simulink model "steady_state_error_test"  (R2017a)
settings: Solver=VariableStepAuto  StartTime=0.0  StopTime=20  RelTol=1e-3
settings Model: Creator=USER  LastModifiedBy=dell

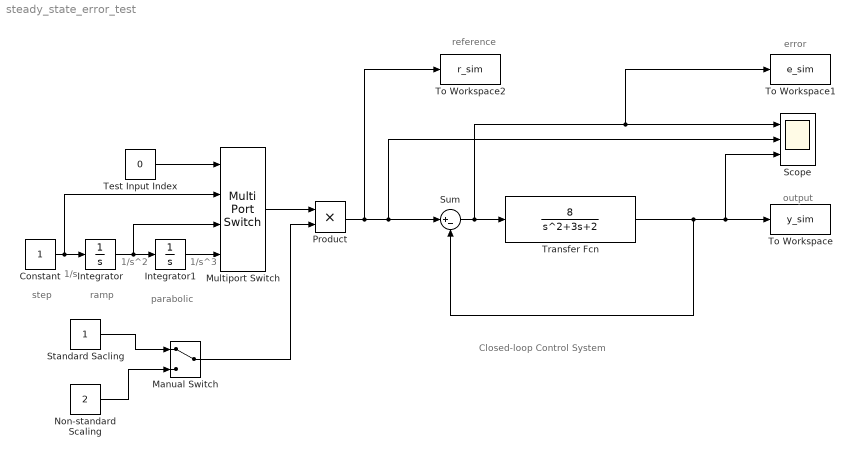
== system steady_state_error_test ==
  note: output
  note: error
  note: reference
  note: parabolic
  note: ramp
  note: step
  note: 1/s^3
  note: 1/s^2
  note: 1/s
  note: Closed-loop Control System
  Constant : Constant
  Integrator : Integrator
  Integrator1 : Integrator
  Manual Switch : ManualSwitch
  Multiport Switch : MultiPortSwitch  DataPortOrder=Zero-based contiguous
  Non-standard Scaling : Constant  Value=2
  Product : Product
  Scope : Scope  NumInputPorts=3
  Standard Sacling : Constant
  Sum : Sum  Inputs=|+-
  Test Input Index : Constant  Value=0
  To Workspace : ToWorkspace  VariableName=y_sim  SaveFormat=Timeseries  SampleTime=-1
  To Workspace1 : ToWorkspace  VariableName=e_sim  SaveFormat=Timeseries  SampleTime=-1
  To Workspace2 : ToWorkspace  VariableName=r_sim  SaveFormat=Timeseries  SampleTime=-1
  Transfer Fcn : TransferFcn  Numerator=[ 8]  Denominator=[1 3 2]
  wires:
  Product/1 -> To Workspace2/1, Sum/1, Scope/2
  Sum/1 -> To Workspace1/1, Scope/1, Transfer Fcn/1
  Transfer Fcn/1 -> Sum/2, To Workspace/1, Scope/3
  Constant/1 -> Integrator/1, Multiport Switch/2
  Integrator/1 -> Integrator1/1, Multiport Switch/3
  Integrator1/1 -> Multiport Switch/4
  Test Input Index/1 -> Multiport Switch/1
  Multiport Switch/1 -> Product/1
  Manual Switch/1 -> Product/2
  Standard Sacling/1 -> Manual Switch/1
  Non-standard Scaling/1 -> Manual Switch/2
